simulink model "FaultMonitoring"  (R2023b)
settings: Solver=VariableStepAuto  StartTime=0.0  StopTime=10.0  RelTol=1e-3
settings Model: Creator=Alkhouly  LastModifiedBy=Alkhouly

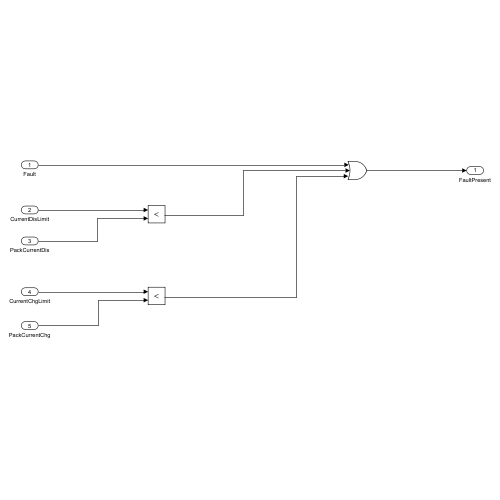
[thumbnail: Simulink's stored preview of the top-level diagram]
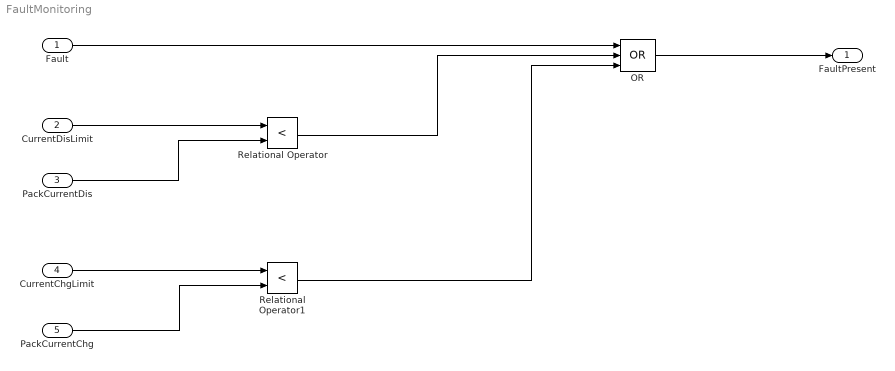
== system FaultMonitoring ==
  Fault : Inport
  CurrentDisLimit : Inport  Port=2
  PackCurrentDis : Inport  Port=3
  CurrentChgLimit : Inport  Port=4
  PackCurrentChg : Inport  Port=5
  OR : Logic  Operator=OR  Inputs=3  IconShape=distinctive  AllPortsSameDT=off  OutDataTypeStr=boolean
  Relational Operator : RelationalOperator  Operator=<  OutDataTypeStr=boolean  RndMeth=Simplest  InputSameDT=off
  Relational Operator1 : RelationalOperator  Operator=<  OutDataTypeStr=boolean  RndMeth=Simplest  InputSameDT=off
  FaultPresent : Outport
  wires:
  Fault/1 -> OR/1
  CurrentDisLimit/1 -> Relational Operator/1
  PackCurrentDis/1 -> Relational Operator/2
  Relational Operator/1 -> OR/2
  Relational Operator1/1 -> OR/3
  CurrentChgLimit/1 -> Relational Operator1/1
  PackCurrentChg/1 -> Relational Operator1/2
  OR/1 -> FaultPresent/1
